simulink model "case2"  (R2024b)
settings: Solver=FixedStepAuto  StartTime=0  StopTime=1  FixedStep=1e-7  RelTol=1e-3
values from neighbouring files (symbols this model uses):
  SG_D_1_D = 0.01056    [IEEE9_case_parameters.m]    (also in case1_parameters.m; case2_parameters.m; case3_parameters.m; case4_parameters.m)
  SG_D_1_EnableSaturation = 0    [IEEE9_case_parameters.m]    (also in case1_parameters.m; case2_parameters.m; case3_parameters.m; case4_parameters.m)
  SG_D_1_f0 = 60    [IEEE9_case_parameters.m]    (also in case1_parameters.m; case2_parameters.m; case3_parameters.m; case4_parameters.m)
  SG_D_1_H = 7.5    [IEEE9_case_parameters.m]    (also in case1_parameters.m; case2_parameters.m; case3_parameters.m; case4_parameters.m)
  SG_D_1_K_A = 20    [IEEE9_case_parameters.m]    (also in case1_parameters.m; case2_parameters.m; case3_parameters.m; case4_parameters.m)
  SG_D_1_K_E = 1.000000e+1    (= 10)    [IEEE9_case_parameters.m]    (also in case1_parameters.m; case2_parameters.m; case3_parameters.m; case4_parameters.m)
  SG_D_1_K_F = 2.363    [IEEE9_case_parameters.m]    (also in case1_parameters.m; case2_parameters.m; case3_parameters.m; case4_parameters.m)
  SG_D_1_K_s = 0.5    [IEEE9_case_parameters.m]    (also in case1_parameters.m = 5; case2_parameters.m = 5; case3_parameters.m = 5; case4_parameters.m = 5)
  SG_D_1_R_a = 0.001088    [IEEE9_case_parameters.m]    (also in case1_parameters.m; case2_parameters.m; case3_parameters.m; case4_parameters.m)
  SG_D_1_S_A = 1    [IEEE9_case_parameters.m]    (also in case1_parameters.m; case2_parameters.m; case3_parameters.m; case4_parameters.m)
  SG_D_1_S_B = 0.103    [IEEE9_case_parameters.m]    (also in case1_parameters.m; case2_parameters.m; case3_parameters.m; case4_parameters.m)
  SG_D_1_S_N = 10.659857    [IEEE9_case_parameters.m]    (also in case1_parameters.m; case2_parameters.m; case3_parameters.m; case4_parameters.m)
  SG_D_1_SpeedPara = 200    [IEEE9_case_parameters.m]    (also in case1_parameters.m; case2_parameters.m; case3_parameters.m; case4_parameters.m)
  SG_D_1_T_0 = 0.720173    [IEEE9_case_parameters.m]    (also in case1_parameters.m = 0.755522; case2_parameters.m = 0.808931; case3_parameters.m = 0.869402; case4_parameters.m = 0.729316)
  SG_D_1_T_1 = 0.3    [IEEE9_case_parameters.m]    (also in case1_parameters.m; case2_parameters.m; case3_parameters.m; case4_parameters.m)
  SG_D_1_T_2 = 0.05    [IEEE9_case_parameters.m]    (also in case1_parameters.m; case2_parameters.m; case3_parameters.m; case4_parameters.m)
  SG_D_1_T_3 = 0.02    [IEEE9_case_parameters.m]    (also in case1_parameters.m; case2_parameters.m; case3_parameters.m; case4_parameters.m)
  SG_D_1_T_4 = 0.005    [IEEE9_case_parameters.m]    (also in case1_parameters.m; case2_parameters.m; case3_parameters.m; case4_parameters.m)
  SG_D_1_T_A = 0.02    [IEEE9_case_parameters.m]    (also in case1_parameters.m; case2_parameters.m; case3_parameters.m; case4_parameters.m)
  SG_D_1_T_dd = 8.000000e+0    (= 8)    [IEEE9_case_parameters.m]    (also in case1_parameters.m; case2_parameters.m; case3_parameters.m; case4_parameters.m)
  SG_D_1_T_ddd = 0.04    [IEEE9_case_parameters.m]    (also in case1_parameters.m; case2_parameters.m; case3_parameters.m; case4_parameters.m)
  SG_D_1_T_E = 0.314    [IEEE9_case_parameters.m]    (also in case1_parameters.m; case2_parameters.m; case3_parameters.m; case4_parameters.m)
  SG_D_1_T_F = 0.35    [IEEE9_case_parameters.m]    (also in case1_parameters.m; case2_parameters.m; case3_parameters.m; case4_parameters.m)
  SG_D_1_T_qd = 0.8    [IEEE9_case_parameters.m]    (also in case1_parameters.m; case2_parameters.m; case3_parameters.m; case4_parameters.m)
  SG_D_1_T_qdd = 0.02    [IEEE9_case_parameters.m]    (also in case1_parameters.m; case2_parameters.m; case3_parameters.m; case4_parameters.m)
  SG_D_1_T_speed = 0.1    [IEEE9_case_parameters.m]    (also in case1_parameters.m = 200; case2_parameters.m = 200; case3_parameters.m = 200; case4_parameters.m = 200)
  SG_D_1_T_w = 0.5    [IEEE9_case_parameters.m]    (also in case1_parameters.m; case2_parameters.m; case3_parameters.m; case4_parameters.m)
  SG_D_1_V_ref = 1.990276    [IEEE9_case_parameters.m]    (also in case1_parameters.m = 2.042296; case2_parameters.m = 2.051388; case3_parameters.m = 2.089584; case4_parameters.m = 2.01845)
  SG_D_1_w_ref = 376.991118    [IEEE9_case_parameters.m]    (also in case1_parameters.m; case2_parameters.m; case3_parameters.m; case4_parameters.m)
  SG_D_1_wb = 6.000000e+1    (= 60)    [IEEE9_case_parameters.m]    (also in case1_parameters.m; case2_parameters.m; case3_parameters.m; case4_parameters.m)
  SG_D_1_x_d = 1.9    [IEEE9_case_parameters.m]    (also in case1_parameters.m; case2_parameters.m; case3_parameters.m; case4_parameters.m)
  SG_D_1_x_dd = 0.302    [IEEE9_case_parameters.m]    (also in case1_parameters.m; case2_parameters.m; case3_parameters.m; case4_parameters.m)
  SG_D_1_x_ddd = 0.204    [IEEE9_case_parameters.m]    (also in case1_parameters.m; case2_parameters.m; case3_parameters.m; case4_parameters.m)
  SG_D_1_x_l = 0.05    [IEEE9_case_parameters.m]    (also in case1_parameters.m; case2_parameters.m; case3_parameters.m; case4_parameters.m)
  SG_D_1_x_q = 1.3    [IEEE9_case_parameters.m]    (also in case1_parameters.m; case2_parameters.m; case3_parameters.m; case4_parameters.m)
  SG_D_1_x_qd = 0.5    [IEEE9_case_parameters.m]    (also in case1_parameters.m; case2_parameters.m; case3_parameters.m; case4_parameters.m)
  SG_D_1_x_qdd = 0.3    [IEEE9_case_parameters.m]    (also in case1_parameters.m; case2_parameters.m; case3_parameters.m; case4_parameters.m)
  SG_D_2_D = 0.02    [IEEE9_case_parameters.m]    (also in case1_parameters.m; case2_parameters.m; case3_parameters.m; case4_parameters.m)
  SG_D_2_EnableSaturation = 0    [IEEE9_case_parameters.m]    (also in case1_parameters.m; case2_parameters.m; case3_parameters.m; case4_parameters.m)
  SG_D_2_f0 = 60    [IEEE9_case_parameters.m]    (also in case1_parameters.m; case2_parameters.m; case3_parameters.m; case4_parameters.m)
  SG_D_2_H = 8.000000e+0    (= 8)    [IEEE9_case_parameters.m]    (also in case1_parameters.m; case2_parameters.m; case3_parameters.m; case4_parameters.m)
  SG_D_2_K_A = 20    [IEEE9_case_parameters.m]    (also in case1_parameters.m; case2_parameters.m; case3_parameters.m; case4_parameters.m)
  SG_D_2_K_E = 1.000000e+1    (= 10)    [IEEE9_case_parameters.m]    (also in case1_parameters.m; case2_parameters.m; case3_parameters.m; case4_parameters.m)
  SG_D_2_K_F = 2.363    [IEEE9_case_parameters.m]    (also in case1_parameters.m; case2_parameters.m; case3_parameters.m; case4_parameters.m)
  SG_D_2_K_s = 0.5    [IEEE9_case_parameters.m]    (also in case1_parameters.m = 4; case2_parameters.m = 4; case3_parameters.m = 4; case4_parameters.m = 4)
  SG_D_2_R_a = 0.001088    [IEEE9_case_parameters.m]    (also in case1_parameters.m; case2_parameters.m; case3_parameters.m; case4_parameters.m)
  SG_D_2_S_A = 1    [IEEE9_case_parameters.m]    (also in case1_parameters.m; case2_parameters.m; case3_parameters.m; case4_parameters.m)
  SG_D_2_S_B = 0.103    [IEEE9_case_parameters.m]    (also in case1_parameters.m; case2_parameters.m; case3_parameters.m; case4_parameters.m)
  SG_D_2_S_N = 10.659857    [IEEE9_case_parameters.m]    (also in case1_parameters.m; case2_parameters.m; case3_parameters.m; case4_parameters.m)
  SG_D_2_SpeedPara = 200    [IEEE9_case_parameters.m]    (also in case1_parameters.m; case2_parameters.m; case3_parameters.m; case4_parameters.m)
  SG_D_2_T_0 = 1.632913    [IEEE9_case_parameters.m]    (also in case1_parameters.m = 1.632925; case2_parameters.m = 1.632915; case3_parameters.m = 1.632914; case4_parameters.m = 1.632927)
  SG_D_2_T_1 = 0.2    [IEEE9_case_parameters.m]    (also in case1_parameters.m; case2_parameters.m; case3_parameters.m; case4_parameters.m)
  SG_D_2_T_2 = 0.05    [IEEE9_case_parameters.m]    (also in case1_parameters.m; case2_parameters.m; case3_parameters.m; case4_parameters.m)
  SG_D_2_T_3 = 0.02    [IEEE9_case_parameters.m]    (also in case1_parameters.m; case2_parameters.m; case3_parameters.m; case4_parameters.m)
  SG_D_2_T_4 = 0.005    [IEEE9_case_parameters.m]    (also in case1_parameters.m; case2_parameters.m; case3_parameters.m; case4_parameters.m)
  SG_D_2_T_A = 0.02    [IEEE9_case_parameters.m]    (also in case1_parameters.m; case2_parameters.m; case3_parameters.m; case4_parameters.m)
  SG_D_2_T_dd = 7.9    [IEEE9_case_parameters.m]    (also in case1_parameters.m; case2_parameters.m; case3_parameters.m; case4_parameters.m)
  SG_D_2_T_ddd = 0.04    [IEEE9_case_parameters.m]    (also in case1_parameters.m; case2_parameters.m; case3_parameters.m; case4_parameters.m)
  SG_D_2_T_E = 0.314    [IEEE9_case_parameters.m]    (also in case1_parameters.m; case2_parameters.m; case3_parameters.m; case4_parameters.m)
  SG_D_2_T_F = 0.35    [IEEE9_case_parameters.m]    (also in case1_parameters.m; case2_parameters.m; case3_parameters.m; case4_parameters.m)
  SG_D_2_T_qd = 0.8    [IEEE9_case_parameters.m]    (also in case1_parameters.m; case2_parameters.m; case3_parameters.m; case4_parameters.m)
  SG_D_2_T_qdd = 0.015    [IEEE9_case_parameters.m]    (also in case1_parameters.m; case2_parameters.m; case3_parameters.m; case4_parameters.m)
  SG_D_2_T_speed = 0.1    [IEEE9_case_parameters.m]    (also in case1_parameters.m = 150; case2_parameters.m = 150; case3_parameters.m = 150; case4_parameters.m = 150)
  SG_D_2_T_w = 0.35    [IEEE9_case_parameters.m]    (also in case1_parameters.m; case2_parameters.m; case3_parameters.m; case4_parameters.m)
  SG_D_2_V_ref = 2.58547    [IEEE9_case_parameters.m]    (also in case1_parameters.m = 2.597896; case2_parameters.m = 2.587136; case3_parameters.m = 2.586042; case4_parameters.m = 2.599679)
  SG_D_2_w_ref = 376.991118    [IEEE9_case_parameters.m]    (also in case1_parameters.m; case2_parameters.m; case3_parameters.m; case4_parameters.m)
  SG_D_2_wb = 6.000000e+1    (= 60)    [IEEE9_case_parameters.m]    (also in case1_parameters.m; case2_parameters.m; case3_parameters.m; case4_parameters.m)
  SG_D_2_x_d = 1.8    [IEEE9_case_parameters.m]    (also in case1_parameters.m; case2_parameters.m; case3_parameters.m; case4_parameters.m)
  SG_D_2_x_dd = 0.302    [IEEE9_case_parameters.m]    (also in case1_parameters.m; case2_parameters.m; case3_parameters.m; case4_parameters.m)
  SG_D_2_x_ddd = 0.204    [IEEE9_case_parameters.m]    (also in case1_parameters.m; case2_parameters.m; case3_parameters.m; case4_parameters.m)
  SG_D_2_x_l = 0.05    [IEEE9_case_parameters.m]    (also in case1_parameters.m; case2_parameters.m; case3_parameters.m; case4_parameters.m)
  SG_D_2_x_q = 1.25    [IEEE9_case_parameters.m]    (also in case1_parameters.m; case2_parameters.m; case3_parameters.m; case4_parameters.m)
  SG_D_2_x_qd = 0.5    [IEEE9_case_parameters.m]    (also in case1_parameters.m; case2_parameters.m; case3_parameters.m; case4_parameters.m)
  SG_D_2_x_qdd = 0.3    [IEEE9_case_parameters.m]    (also in case1_parameters.m; case2_parameters.m; case3_parameters.m; case4_parameters.m)
  SG_D_3_D = 0.02    [IEEE9_case_parameters.m]    (also in case1_parameters.m; case2_parameters.m; case3_parameters.m; case4_parameters.m)
  SG_D_3_EnableSaturation = 0    [IEEE9_case_parameters.m]    (also in case1_parameters.m; case2_parameters.m; case3_parameters.m; case4_parameters.m)
  SG_D_3_f0 = 60    [IEEE9_case_parameters.m]    (also in case1_parameters.m; case2_parameters.m; case3_parameters.m; case4_parameters.m)
  SG_D_3_H = 7.7    [IEEE9_case_parameters.m]    (also in case1_parameters.m; case2_parameters.m; case3_parameters.m; case4_parameters.m)
  SG_D_3_K_A = 20    [IEEE9_case_parameters.m]    (also in case1_parameters.m; case2_parameters.m; case3_parameters.m; case4_parameters.m)
  SG_D_3_K_E = 1.000000e+1    (= 10)    [IEEE9_case_parameters.m]    (also in case1_parameters.m; case2_parameters.m; case3_parameters.m; case4_parameters.m)
  SG_D_3_K_F = 2.363    [IEEE9_case_parameters.m]    (also in case1_parameters.m; case2_parameters.m; case3_parameters.m; case4_parameters.m)
  SG_D_3_K_s = 0.2    [IEEE9_case_parameters.m]    (also in case1_parameters.m = 2; case2_parameters.m = 2; case3_parameters.m = 2; case4_parameters.m = 2)
  SG_D_3_R_a = 0.001088    [IEEE9_case_parameters.m]    (also in case1_parameters.m; case2_parameters.m; case3_parameters.m; case4_parameters.m)
  SG_D_3_S_A = 1    [IEEE9_case_parameters.m]    (also in case1_parameters.m; case2_parameters.m; case3_parameters.m; case4_parameters.m)
  SG_D_3_S_B = 0.103    [IEEE9_case_parameters.m]    (also in case1_parameters.m; case2_parameters.m; case3_parameters.m; case4_parameters.m)
  SG_D_3_S_N = 10.659857    [IEEE9_case_parameters.m]    (also in case1_parameters.m; case2_parameters.m; case3_parameters.m; case4_parameters.m)
  SG_D_3_SpeedPara = 200    [IEEE9_case_parameters.m]    (also in case1_parameters.m; case2_parameters.m; case3_parameters.m; case4_parameters.m)
  SG_D_3_T_0 = 0.850788    [IEEE9_case_parameters.m]    (also in case1_parameters.m = 0.850786; case2_parameters.m = 0.850787; case3_parameters.m; case4_parameters.m = 0.850786)
  SG_D_3_T_1 = 0.2    [IEEE9_case_parameters.m]    (also in case1_parameters.m; case2_parameters.m; case3_parameters.m; case4_parameters.m)
  SG_D_3_T_2 = 0.05    [IEEE9_case_parameters.m]    (also in case1_parameters.m; case2_parameters.m; case3_parameters.m; case4_parameters.m)
  SG_D_3_T_3 = 0.02    [IEEE9_case_parameters.m]    (also in case1_parameters.m; case2_parameters.m; case3_parameters.m; case4_parameters.m)
  SG_D_3_T_4 = 0.005    [IEEE9_case_parameters.m]    (also in case1_parameters.m; case2_parameters.m; case3_parameters.m; case4_parameters.m)
  SG_D_3_T_A = 0.02    [IEEE9_case_parameters.m]    (also in case1_parameters.m; case2_parameters.m; case3_parameters.m; case4_parameters.m)
  SG_D_3_T_dd = 8.1    [IEEE9_case_parameters.m]    (also in case1_parameters.m; case2_parameters.m; case3_parameters.m; case4_parameters.m)
  SG_D_3_T_ddd = 0.04    [IEEE9_case_parameters.m]    (also in case1_parameters.m; case2_parameters.m; case3_parameters.m; case4_parameters.m)
  SG_D_3_T_E = 0.314    [IEEE9_case_parameters.m]    (also in case1_parameters.m; case2_parameters.m; case3_parameters.m; case4_parameters.m)
  SG_D_3_T_F = 0.35    [IEEE9_case_parameters.m]    (also in case1_parameters.m; case2_parameters.m; case3_parameters.m; case4_parameters.m)
  SG_D_3_T_qd = 0.8    [IEEE9_case_parameters.m]    (also in case1_parameters.m; case2_parameters.m; case3_parameters.m; case4_parameters.m)
  SG_D_3_T_qdd = 0.015    [IEEE9_case_parameters.m]    (also in case1_parameters.m; case2_parameters.m; case3_parameters.m; case4_parameters.m)
  SG_D_3_T_speed = 0.1    [IEEE9_case_parameters.m]    (also in case1_parameters.m = 180; case2_parameters.m = 180; case3_parameters.m = 180; case4_parameters.m = 180)
  SG_D_3_T_w = 0.4    [IEEE9_case_parameters.m]    (also in case1_parameters.m; case2_parameters.m; case3_parameters.m; case4_parameters.m)
  SG_D_3_V_ref = 1.892727    [IEEE9_case_parameters.m]    (also in case1_parameters.m = 1.906439; case2_parameters.m = 1.895535; case3_parameters.m = 1.892105; case4_parameters.m = 1.906598)
  SG_D_3_w_ref = 376.991118    [IEEE9_case_parameters.m]    (also in case1_parameters.m; case2_parameters.m; case3_parameters.m; case4_parameters.m)
  SG_D_3_wb = 6.000000e+1    (= 60)    [IEEE9_case_parameters.m]    (also in case1_parameters.m; case2_parameters.m; case3_parameters.m; case4_parameters.m)
  SG_D_3_x_d = 1.85    [IEEE9_case_parameters.m]    (also in case1_parameters.m; case2_parameters.m; case3_parameters.m; case4_parameters.m)
  SG_D_3_x_dd = 0.302    [IEEE9_case_parameters.m]    (also in case1_parameters.m; case2_parameters.m; case3_parameters.m; case4_parameters.m)
  SG_D_3_x_ddd = 0.204    [IEEE9_case_parameters.m]    (also in case1_parameters.m; case2_parameters.m; case3_parameters.m; case4_parameters.m)
  SG_D_3_x_l = 0.05    [IEEE9_case_parameters.m]    (also in case1_parameters.m; case2_parameters.m; case3_parameters.m; case4_parameters.m)
  SG_D_3_x_q = 1.2    [IEEE9_case_parameters.m]    (also in case1_parameters.m; case2_parameters.m; case3_parameters.m; case4_parameters.m)
  SG_D_3_x_qd = 0.5    [IEEE9_case_parameters.m]    (also in case1_parameters.m; case2_parameters.m; case3_parameters.m; case4_parameters.m)
  SG_D_3_x_qdd = 0.3    [IEEE9_case_parameters.m]    (also in case1_parameters.m; case2_parameters.m; case3_parameters.m; case4_parameters.m)
(part 1 of 12)
settings Model: Creator=Greg  LastModifiedBy=Greg

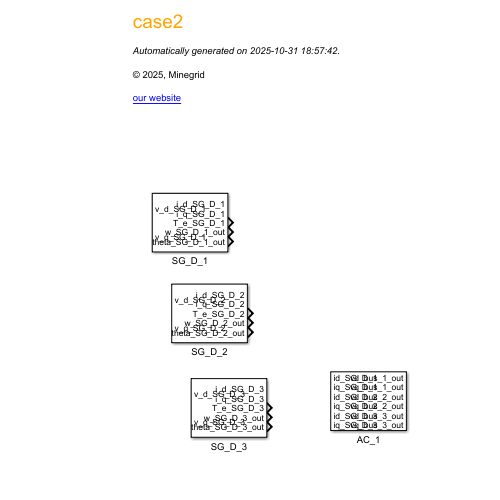
[thumbnail: Simulink's stored preview of the top-level diagram]
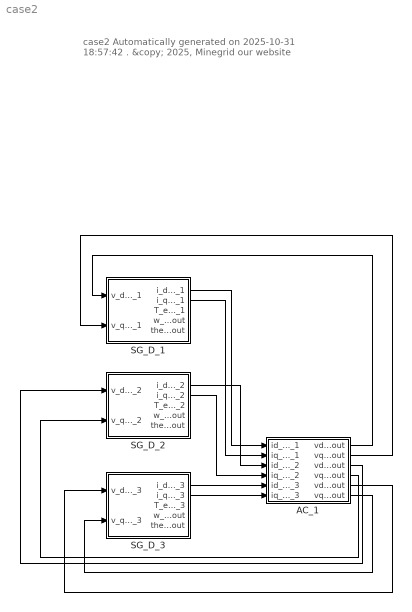
== system case2 ==
  note: case2
      | Automatically generated on 2025-10-31 18:57:42 .
      | &copy; 2025, Minegrid
      | our website
  AC_1 : Subsystem  mask(AC_1){}
      mask help: Parameters Interface of AC_1
  SG_D_1 : Subsystem  mask(SG_D_1){T_0=SG_D_1_T_0, w_ref=SG_D_1_w_ref, V_ref=SG_D_1_V_ref, x_d=SG_D_1_x_d, x_dd=SG_D_1_x_dd, x_ddd=SG_D_1_x_ddd, x_q=SG_D_1_x_q, x_qd=SG_D_1_x_qd, x_qdd=SG_D_1_x_qdd, x_l=SG_D_1_x_l, R_a=SG_D_1_R_a, T_dd=SG_D_1_T_dd, T_ddd=SG_D_1_T_ddd, T_qd=SG_D_1_T_qd, T_qdd=SG_D_1_T_qdd, H=SG_D_1_H, D=SG_D_1_D, SpeedPara=SG_D_1_SpeedPara, K_A=SG_D_1_K_A, EnableSaturation=SG_D_1_EnableSaturation, f0=SG_D_1_f0, T_speed=SG_D_1_T_speed, T_E=SG_D_1_T_E, T_A=SG_D_1_T_A, T_F=SG_D_1_T_F, K_E=SG_D_1_K_E, K_F=SG_D_1_K_F, K_s=SG_D_1_K_s, T_1=SG_D_1_T_1, T_2=SG_D_1_T_2, T_3=SG_D_1_T_3, T_4=SG_D_1_T_4, T_w=SG_D_1_T_w, wb=SG_D_1_wb, S_A=SG_D_1_S_A, S_B=SG_D_1_S_B, S_N=SG_D_1_S_N}
      mask help: Parameters Interface of SG_D_1
  SG_D_2 : Subsystem  mask(SG_D_2){T_0=SG_D_2_T_0, w_ref=SG_D_2_w_ref, V_ref=SG_D_2_V_ref, x_d=SG_D_2_x_d, x_dd=SG_D_2_x_dd, x_ddd=SG_D_2_x_ddd, x_q=SG_D_2_x_q, x_qd=SG_D_2_x_qd, x_qdd=SG_D_2_x_qdd, x_l=SG_D_2_x_l, R_a=SG_D_2_R_a, T_dd=SG_D_2_T_dd, T_ddd=SG_D_2_T_ddd, T_qd=SG_D_2_T_qd, T_qdd=SG_D_2_T_qdd, H=SG_D_2_H, D=SG_D_2_D, SpeedPara=SG_D_2_SpeedPara, K_A=SG_D_2_K_A, EnableSaturation=SG_D_2_EnableSaturation, f0=SG_D_2_f0, T_speed=SG_D_2_T_speed, T_E=SG_D_2_T_E, T_A=SG_D_2_T_A, T_F=SG_D_2_T_F, K_E=SG_D_2_K_E, K_F=SG_D_2_K_F, K_s=SG_D_2_K_s, T_1=SG_D_2_T_1, T_2=SG_D_2_T_2, T_3=SG_D_2_T_3, T_4=SG_D_2_T_4, T_w=SG_D_2_T_w, wb=SG_D_2_wb, S_A=SG_D_2_S_A, S_B=SG_D_2_S_B, S_N=SG_D_2_S_N}
      mask help: Parameters Interface of SG_D_2
  SG_D_3 : Subsystem  mask(SG_D_3){T_0=SG_D_3_T_0, w_ref=SG_D_3_w_ref, V_ref=SG_D_3_V_ref, x_d=SG_D_3_x_d, x_dd=SG_D_3_x_dd, x_ddd=SG_D_3_x_ddd, x_q=SG_D_3_x_q, x_qd=SG_D_3_x_qd, x_qdd=SG_D_3_x_qdd, x_l=SG_D_3_x_l, R_a=SG_D_3_R_a, T_dd=SG_D_3_T_dd, T_ddd=SG_D_3_T_ddd, T_qd=SG_D_3_T_qd, T_qdd=SG_D_3_T_qdd, H=SG_D_3_H, D=SG_D_3_D, SpeedPara=SG_D_3_SpeedPara, K_A=SG_D_3_K_A, EnableSaturation=SG_D_3_EnableSaturation, f0=SG_D_3_f0, T_speed=SG_D_3_T_speed, T_E=SG_D_3_T_E, T_A=SG_D_3_T_A, T_F=SG_D_3_T_F, K_E=SG_D_3_K_E, K_F=SG_D_3_K_F, K_s=SG_D_3_K_s, T_1=SG_D_3_T_1, T_2=SG_D_3_T_2, T_3=SG_D_3_T_3, T_4=SG_D_3_T_4, T_w=SG_D_3_T_w, wb=SG_D_3_wb, S_A=SG_D_3_S_A, S_B=SG_D_3_S_B, S_N=SG_D_3_S_N}
      mask help: Parameters Interface of SG_D_3
  wires:
  SG_D_2/2(i_q_SG_D_2) -> AC_1/4(iq_SG_D_2)
  SG_D_1/2(i_q_SG_D_1) -> AC_1/2(iq_SG_D_1)
  SG_D_1/1(i_d_SG_D_1) -> AC_1/1(id_SG_D_1)
  SG_D_2/1(i_d_SG_D_2) -> AC_1/3(id_SG_D_2)
  AC_1/1(vd_bus_1_out) -> SG_D_1/1(v_d_SG_D_1)
  SG_D_3/1(i_d_SG_D_3) -> AC_1/5(id_SG_D_3)
  AC_1/2(vq_bus_1_out) -> SG_D_1/2(v_q_SG_D_1)
  SG_D_3/2(i_q_SG_D_3) -> AC_1/6(iq_SG_D_3)
  AC_1/3(vd_bus_2_out) -> SG_D_2/1(v_d_SG_D_2)
  AC_1/4(vq_bus_2_out) -> SG_D_2/2(v_q_SG_D_2)
  AC_1/5(vd_bus_3_out) -> SG_D_3/1(v_d_SG_D_3)
  AC_1/6(vq_bus_3_out) -> SG_D_3/2(v_q_SG_D_3)

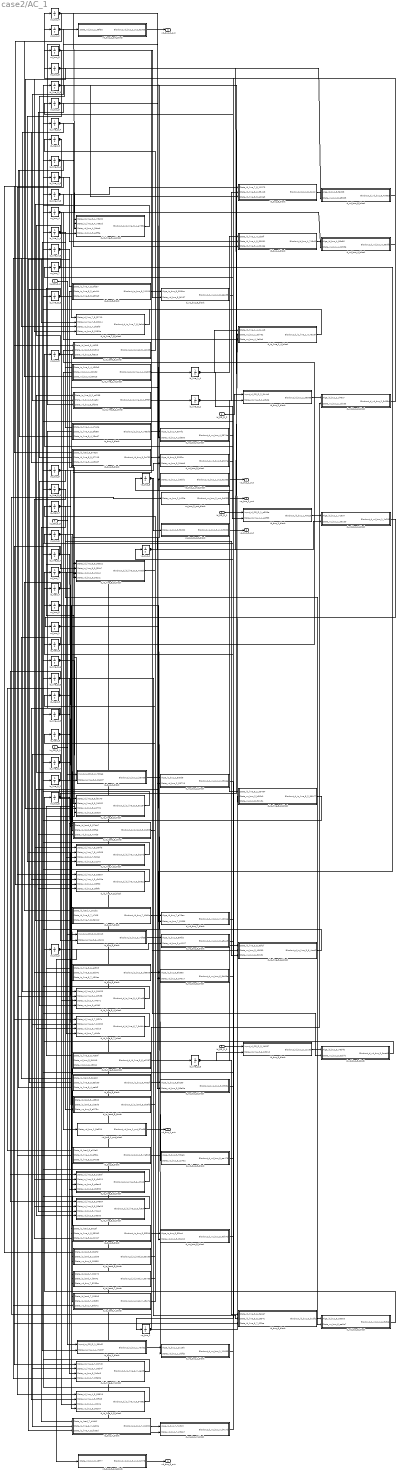
== system case2/AC_1 ==
  id_SG_D_1 : Inport
  iq_SG_D_1 : Inport  Port=2
  id_SG_D_2 : Inport  Port=3
  iq_SG_D_2 : Inport  Port=4
  id_SG_D_3 : Inport  Port=5
  iq_SG_D_3 : Inport  Port=6
  d_id_line_1_4_block : Subsystem
  d_id_line_3_6_block : Subsystem
  d_id_line_4_5_block : Subsystem
  d_id_line_5_6_block : Subsystem
  d_id_line_6_7_block : Subsystem
  d_id_line_7_8_block : Subsystem
  d_id_line_8_2_block : Subsystem
  d_id_line_8_9_block : Subsystem
  d_id_line_9_4_block : Subsystem
  d_id_load_5_block : Subsystem
  d_id_load_7_block : Subsystem
  d_id_load_9_block : Subsystem
  d_iq_line_1_4_block : Subsystem
  d_iq_line_3_6_block : Subsystem
  d_iq_line_4_5_block : Subsystem
  d_iq_line_5_6_block : Subsystem
  d_iq_line_6_7_block : Subsystem
  d_iq_line_7_8_block : Subsystem
  d_iq_line_8_2_block : Subsystem
  d_iq_line_8_9_block : Subsystem
  d_iq_line_9_4_block : Subsystem
  d_iq_load_5_block : Subsystem
  d_iq_load_7_block : Subsystem
  d_iq_load_9_block : Subsystem
  d_vd_bus_1_block : Subsystem
  d_vd_bus_2_block : Subsystem
  d_vd_bus_3_block : Subsystem
  d_vd_bus_4_block : Subsystem
  d_vd_bus_5_block : Subsystem
  d_vd_bus_6_block : Subsystem
  d_vd_bus_7_block : Subsystem
  d_vd_bus_8_block : Subsystem
  d_vd_bus_9_block : Subsystem
  d_vq_bus_1_block : Subsystem
  d_vq_bus_2_block : Subsystem
  d_vq_bus_3_block : Subsystem
  d_vq_bus_4_block : Subsystem
  d_vq_bus_5_block : Subsystem
  d_vq_bus_6_block : Subsystem
  d_vq_bus_7_block : Subsystem
  d_vq_bus_8_block : Subsystem
  d_vq_bus_9_block : Subsystem
  id_bus_1_block : Subsystem
  id_bus_2_block : Subsystem
  id_bus_3_block : Subsystem
  id_bus_4_block : Subsystem
  id_bus_5_block : Subsystem
  id_bus_6_block : Subsystem
  id_bus_7_block : Subsystem
  id_bus_8_block : Subsystem
  id_bus_9_block : Subsystem
  id_line_1_4 : Integrator  InitialCondition=0.8082
  id_line_3_6 : Integrator  InitialCondition=0.8457
  id_line_4_5 : Integrator  InitialCondition=0.3479
  id_line_5_6 : Integrator  InitialCondition=-0.5937
  id_line_6_7 : Integrator  InitialCondition=0.2581
  id_line_7_8 : Integrator  InitialCondition=-0.7857
  id_line_8_2 : Integrator  InitialCondition=-1.6336
  id_line_8_9 : Integrator  InitialCondition=0.8599
  id_line_9_4 : Integrator  InitialCondition=-0.4527
  id_load_5 : Integrator  InitialCondition=0.9220949046655532
  id_load_7 : Integrator  InitialCondition=1.043451181339317
  id_load_9 : Integrator  InitialCondition=1.2932545562048015
  iq_bus_1_block : Subsystem
  iq_bus_2_block : Subsystem
  iq_bus_3_block : Subsystem
  iq_bus_4_block : Subsystem
  iq_bus_5_block : Subsystem
  iq_bus_6_block : Subsystem
  iq_bus_7_block : Subsystem
  iq_bus_8_block : Subsystem
  iq_bus_9_block : Subsystem
  iq_line_1_4 : Integrator  InitialCondition=-0.2445
  iq_line_3_6 : Integrator  InitialCondition=0.0905
  iq_line_4_5 : Integrator  InitialCondition=-0.0855
  iq_line_5_6 : Integrator  InitialCondition=0.0474
  iq_line_6_7 : Integrator  InitialCondition=-0.1464
  iq_line_7_8 : Integrator  InitialCondition=0.0394
  iq_line_8_2 : Integrator  InitialCondition=-0.1018
  iq_line_8_9 : Integrator  InitialCondition=-0.0851
  iq_line_9_4 : Integrator  InitialCondition=0.3237
  iq_load_5 : Integrator  InitialCondition=-0.3839325127306236
  iq_load_7 : Integrator  InitialCondition=-0.3621433932821941
  iq_load_9 : Integrator  InitialCondition=-0.6389217940515789
  vd_bus_1 : Integrator  InitialCondition=1.0
  vd_bus_1_out_block : Subsystem
  vd_bus_2 : Integrator  InitialCondition=0.9882467673333026
  vd_bus_2_out_block : Subsystem
  vd_bus_3 : Integrator  InitialCondition=0.9975390275639218
  vd_bus_3_out_block : Subsystem
  vd_bus_4 : Integrator  InitialCondition=0.9862000078347533
  vd_bus_5 : Integrator  InitialCondition=0.9728788660812012
  vd_bus_6 : Integrator  InitialCondition=1.0027357442532745
  vd_bus_7 : Integrator  InitialCondition=0.9853647003996387
  vd_bus_8 : Integrator  InitialCondition=0.9944780823647019
  vd_bus_9 : Integrator  InitialCondition=0.9549499810613831
  vq_bus_1 : Integrator  InitialCondition=0.0
  vq_bus_1_out_block : Subsystem
  vq_bus_2 : Integrator  InitialCondition=0.1528670234395801
  vq_bus_2_out_block : Subsystem
  vq_bus_3 : Integrator  InitialCondition=0.07011339734191536
  vq_bus_3_out_block : Subsystem
  vq_bus_4 : Integrator  InitialCondition=-0.04560902069175053
  vq_bus_5 : Integrator  InitialCondition=-0.07558645534686588
  vq_bus_6 : Integrator  InitialCondition=0.021554874164418644
  vq_bus_7 : Integrator  InitialCondition=-0.002285093510706759
  vq_bus_8 : Integrator  InitialCondition=0.05282760910237743
  vq_bus_9 : Integrator  InitialCondition=-0.08023822590177464
  vd_bus_1_out : Outport
  vq_bus_1_out : Outport  Port=2
  vd_bus_2_out : Outport  Port=3
  vq_bus_2_out : Outport  Port=4
  vd_bus_3_out : Outport  Port=5
  vq_bus_3_out : Outport  Port=6
  wires:
  iq_SG_D_2/1 -> iq_bus_2_block/1(Input_iq_SG_D_2_708e6)
  id_bus_4_block/1(Blockout_id_bus_4_748d0) -> d_vd_bus_4_block/1(Alge_id_bus_4_86c66)
  vd_bus_1_out_block/1(Blockout_vd_bus_1_out_57e66) -> vd_bus_1_out/1
  vq_bus_1_out_block/1(Blockout_vq_bus_1_out_5135a) -> vq_bus_1_out/1
  id_load_9/1 -> d_id_load_9_block/1(State_id_load_9_4df15), id_bus_9_block/1(State_id_load_9_97526), d_iq_load_9_block/1(State_id_load_9_3b2fd)
  vq_bus_2_out_block/1(Blockout_vq_bus_2_out_0c630) -> vq_bus_2_out/1
  d_id_line_1_4_block/1(Blockout_d_id_line_1_4_0ab3f) -> id_line_1_4/1
  iq_SG_D_3/1 -> iq_bus_3_block/1(Input_iq_SG_D_3_22043)
  vq_bus_1/1 -> d_vd_bus_1_block/2(State_vq_bus_1_a61e0), vq_bus_1_out_block/1(State_vq_bus_1_b3dd1), d_iq_line_1_4_block/2(State_vq_bus_1_ed792)
  vd_bus_3_out_block/1(Blockout_vd_bus_3_out_24978) -> vd_bus_3_out/1
  d_vd_bus_4_block/1(Blockout_d_vd_bus_4_39df0) -> vd_bus_4/1
  d_iq_line_8_2_block/1(Blockout_d_iq_line_8_2_96b77) -> iq_line_8_2/1
  id_SG_D_3/1 -> id_bus_3_block/1(Input_id_SG_D_3_1b557)
  id_bus_9_block/1(Blockout_id_bus_9_2e79f) -> d_vd_bus_9_block/1(Alge_id_bus_9_3932a)
  iq_SG_D_1/1 -> iq_bus_1_block/1(Input_iq_SG_D_1_56b6f)
  iq_bus_2_block/1(Blockout_iq_bus_2_b5069) -> d_vq_bus_2_block/1(Alge_iq_bus_2_5c6d8)
  vd_bus_6/1 -> d_vq_bus_6_block/2(State_vd_bus_6_e4a17), d_id_line_3_6_block/3(State_vd_bus_6_1884c), d_id_line_6_7_block/3(State_vd_bus_6_7ad19), d_id_line_5_6_block/4(State_vd_bus_6_a9a0a)
  d_id_line_4_5_block/1(Blockout_d_id_line_4_5_ba811) -> id_line_4_5/1
  vq_bus_2/1 -> d_iq_line_8_2_block/2(State_vq_bus_2_b36b0), d_vd_bus_2_block/2(State_vq_bus_2_1d16a), vq_bus_2_out_block/1(State_vq_bus_2_b12fe)
  id_SG_D_2/1 -> id_bus_2_block/1(Input_id_SG_D_2_544c5)
  id_SG_D_1/1 -> id_bus_1_block/1(Input_id_SG_D_1_a599e)
  iq_bus_4_block/1(Blockout_iq_bus_4_79ed0) -> d_vq_bus_4_block/1(Alge_iq_bus_4_697f2)
  id_line_6_7/1 -> d_id_line_6_7_block/1(State_id_line_6_7_5f97c), d_iq_line_6_7_block/1(State_id_line_6_7_327c8), id_bus_6_block/3(State_id_line_6_7_02fca), id_bus_7_block/2(State_id_line_6_7_c74f6)
  id_bus_2_block/1(Blockout_id_bus_2_a8585) -> d_vd_bus_2_block/1(Alge_id_bus_2_d46c7)
  vq_bus_7/1 -> d_vd_bus_7_block/2(State_vq_bus_7_81f66), d_iq_line_7_8_block/3(State_vq_bus_7_5bef0), d_iq_line_6_7_block/4(State_vq_bus_7_35686), d_iq_load_7_block/3(State_vq_bus_7_90b72)
  vd_bus_2_out_block/1(Blockout_vd_bus_2_out_3230a) -> vd_bus_2_out/1
  iq_bus_9_block/1(Blockout_iq_bus_9_46ecf) -> d_vq_bus_9_block/1(Alge_iq_bus_9_5bc50)
  vq_bus_3_out_block/1(Blockout_vq_bus_3_out_fc8db) -> vq_bus_3_out/1
  iq_bus_8_block/1(Blockout_iq_bus_8_11109) -> d_vq_bus_8_block/1(Alge_iq_bus_8_0994e)
  d_id_line_6_7_block/1(Blockout_d_id_line_6_7_9dd44) -> id_line_6_7/1
  d_iq_line_9_4_block/1(Blockout_d_iq_line_9_4_61cd6) -> iq_line_9_4/1
  id_line_5_6/1 -> d_id_line_5_6_block/1(State_id_line_5_6_54864), d_iq_line_5_6_block/1(State_id_line_5_6_a16ef), id_bus_5_block/3(State_id_line_5_6_04a55), id_bus_6_block/2(State_id_line_5_6_c534c)
  id_bus_3_block/1(Blockout_id_bus_3_1118d) -> d_vd_bus_3_block/1(Alge_id_bus_3_78d4b)
  id_bus_8_block/1(Blockout_id_bus_8_d4ccc) -> d_vd_bus_8_block/1(Alge_id_bus_8_f6d08)
  iq_bus_7_block/1(Blockout_iq_bus_7_1b282) -> d_vq_bus_7_block/1(Alge_iq_bus_7_7a913)
  iq_bus_1_block/1(Blockout_iq_bus_1_79d62) -> d_vq_bus_1_block/1(Alge_iq_bus_1_2119b)
  id_bus_7_block/1(Blockout_id_bus_7_4fd6a) -> d_vd_bus_7_block/1(Alge_id_bus_7_e76ec)
  d_id_load_7_block/1(Blockout_d_id_load_7_5a75a) -> id_load_7/1
  iq_bus_6_block/1(Blockout_iq_bus_6_d8605) -> d_vq_bus_6_block/1(Alge_iq_bus_6_8b56a)
  id_line_4_5/1 -> id_bus_4_block/2(State_id_line_4_5_50091), d_iq_line_4_5_block/1(State_id_line_4_5_89819), d_id_line_4_5_block/1(State_id_line_4_5_63ee7), id_bus_5_block/2(State_id_line_4_5_6f8c4)
  id_bus_6_block/1(Blockout_id_bus_6_b1df2) -> d_vd_bus_6_block/1(Alge_id_bus_6_030aa)
  iq_bus_5_block/1(Blockout_iq_bus_5_9f39d) -> d_vq_bus_5_block/1(Alge_iq_bus_5_8f4e4)
  id_bus_5_block/1(Blockout_id_bus_5_7e5b8) -> d_vd_bus_5_block/1(Alge_id_bus_5_78beb)
  iq_bus_3_block/1(Blockout_iq_bus_3_7dfe9) -> d_vq_bus_3_block/1(Alge_iq_bus_3_59f2b)
  iq_line_9_4/1 -> d_id_line_9_4_block/2(State_iq_line_9_4_7582d), d_iq_line_9_4_block/2(State_iq_line_9_4_bf158), iq_bus_4_block/3(State_iq_line_9_4_15ad7), iq_bus_9_block/3(State_iq_line_9_4_aebff)
  d_iq_line_3_6_block/1(Blockout_d_iq_line_3_6_4acdf) -> iq_line_3_6/1
  vd_bus_4/1 -> d_id_line_1_4_block/3(State_vd_bus_4_b081e), d_id_line_4_5_block/3(State_vd_bus_4_38f30), d_id_line_9_4_block/3(State_vd_bus_4_3cbcb), d_vq_bus_4_block/2(State_vd_bus_4_2d95a)
  id_line_9_4/1 -> d_id_line_9_4_block/1(State_id_line_9_4_78432), d_iq_line_9_4_block/1(State_id_line_9_4_54433), id_bus_4_block/3(State_id_line_9_4_0046a), id_bus_9_block/3(State_id_line_9_4_b960f)
  vq_bus_8/1 -> d_iq_line_8_2_block/3(State_vq_bus_8_91184), d_iq_line_7_8_block/4(State_vq_bus_8_9183e), d_vd_bus_8_block/2(State_vq_bus_8_658d5), d_iq_line_8_9_block/3(State_vq_bus_8_a2731)
  d_vq_bus_8_block/1(Blockout_d_vq_bus_8_66a55) -> vq_bus_8/1
  id_load_7/1 -> id_bus_7_block/1(State_id_load_7_161b2), d_iq_load_7_block/1(State_id_load_7_916b5), d_id_load_7_block/1(State_id_load_7_50270)
  id_line_1_4/1 -> d_iq_line_1_4_block/1(State_id_line_1_4_24448), id_bus_4_block/1(State_id_line_1_4_2b5ff), id_bus_1_block/2(State_id_line_1_4_e0f83)
  id_bus_1_block/1(Blockout_id_bus_1_49cc3) -> d_vd_bus_1_block/1(Alge_id_bus_1_716c4)
  d_iq_line_6_7_block/1(Blockout_d_iq_line_6_7_4ed8f) -> iq_line_6_7/1
  d_vd_bus_7_block/1(Blockout_d_vd_bus_7_1b34a) -> vd_bus_7/1
  vd_bus_9/1 -> d_vq_bus_9_block/2(State_vd_bus_9_96e3e), d_id_load_9_block/3(State_vd_bus_9_f0529), d_id_line_8_9_block/4(State_vd_bus_9_a61c1), d_id_line_9_4_block/4(State_vd_bus_9_e3f3e)
  d_id_line_8_2_block/1(Blockout_d_id_line_8_2_9ff87) -> id_line_8_2/1
  d_vq_bus_9_block/1(Blockout_d_vq_bus_9_3fd84) -> vq_bus_9/1
  iq_load_9/1 -> d_id_load_9_block/2(State_iq_load_9_81910), d_iq_load_9_block/2(State_iq_load_9_12d39), iq_bus_9_block/1(State_iq_load_9_0a6dd)
  vd_bus_2/1 -> d_vq_bus_2_block/2(State_vd_bus_2_59719), vd_bus_2_out_block/1(State_vd_bus_2_38fae), d_id_line_8_2_block/2(State_vd_bus_2_94e9c)
  d_id_line_3_6_block/1(Blockout_d_id_line_3_6_a1287) -> id_line_3_6/1
  vd_bus_7/1 -> d_vq_bus_7_block/2(State_vd_bus_7_25da7), d_id_line_6_7_block/4(State_vd_bus_7_c0c3c), d_id_line_7_8_block/3(State_vd_bus_7_f48ac), d_id_load_7_block/3(State_vd_bus_7_8233e)
  iq_load_5/1 -> d_id_load_5_block/2(State_iq_load_5_85fa6), iq_bus_5_block/1(State_iq_load_5_a6c3f), d_iq_load_5_block/2(State_iq_load_5_1b5d6)
  id_line_8_9/1 -> id_bus_8_block/3(State_id_line_8_9_a20e3), d_id_line_8_9_block/1(State_id_line_8_9_36022), d_iq_line_8_9_block/1(State_id_line_8_9_f0140), id_bus_9_block/2(State_id_line_8_9_07115)
  vd_bus_3/1 -> d_vq_bus_3_block/2(State_vd_bus_3_a1107), d_id_line_3_6_block/2(State_vd_bus_3_54849), vd_bus_3_out_block/1(State_vd_bus_3_18f77)
  id_line_8_2/1 -> d_iq_line_8_2_block/1(State_id_line_8_2_ae494), id_bus_8_block/2(State_id_line_8_2_95418), id_bus_2_block/2(State_id_line_8_2_af6d6)
  iq_line_7_8/1 -> d_id_line_7_8_block/2(State_iq_line_7_8_44268), d_iq_line_7_8_block/2(State_iq_line_7_8_8dc14), iq_bus_7_block/3(State_iq_line_7_8_f10ed), iq_bus_8_block/1(State_iq_line_7_8_0fde7)
  iq_line_4_5/1 -> d_iq_line_4_5_block/2(State_iq_line_4_5_9f9c8), iq_bus_4_block/2(State_iq_line_4_5_efb88), iq_bus_5_block/2(State_iq_line_4_5_553d2), d_id_line_4_5_block/2(State_iq_line_4_5_db19e)
  iq_line_8_9/1 -> d_id_line_8_9_block/2(State_iq_line_8_9_f99c7), d_iq_line_8_9_block/2(State_iq_line_8_9_2d182), iq_bus_8_block/3(State_iq_line_8_9_635a9), iq_bus_9_block/2(State_iq_line_8_9_83b30)
  vd_bus_8/1 -> d_vq_bus_8_block/2(State_vd_bus_8_fb157), d_id_line_7_8_block/4(State_vd_bus_8_1c270), d_id_line_8_9_block/3(State_vd_bus_8_d11ac), d_id_line_8_2_block/3(State_vd_bus_8_dfb0e)
  iq_line_5_6/1 -> d_id_line_5_6_block/2(State_iq_line_5_6_98e26), iq_bus_5_block/3(State_iq_line_5_6_211b7), iq_bus_6_block/2(State_iq_line_5_6_6d34c), d_iq_line_5_6_block/2(State_iq_line_5_6_db011)
  iq_line_8_2/1 -> d_id_line_8_2_block/1(State_iq_line_8_2_cd298), iq_bus_2_block/2(State_iq_line_8_2_8ad2f), iq_bus_8_block/2(State_iq_line_8_2_e4d44)
  id_line_7_8/1 -> id_bus_8_block/1(State_id_line_7_8_11373), d_id_line_7_8_block/1(State_id_line_7_8_397f6), d_iq_line_7_8_block/1(State_id_line_7_8_f0710), id_bus_7_block/3(State_id_line_7_8_561bd)
  iq_line_6_7/1 -> d_id_line_6_7_block/2(State_iq_line_6_7_b228d), d_iq_line_6_7_block/2(State_iq_line_6_7_06b4f), iq_bus_6_block/3(State_iq_line_6_7_450ec), iq_bus_7_block/2(State_iq_line_6_7_cab3a)
  id_line_3_6/1 -> d_iq_line_3_6_block/1(State_id_line_3_6_9bf1f), id_bus_3_block/2(State_id_line_3_6_b321d), id_bus_6_block/1(State_id_line_3_6_3a667)
  iq_line_3_6/1 -> d_id_line_3_6_block/1(State_iq_line_3_6_4c99f), iq_bus_3_block/2(State_iq_line_3_6_4d41b), iq_bus_6_block/1(State_iq_line_3_6_ec9b9)
  vq_bus_9/1 -> d_vd_bus_9_block/2(State_vq_bus_9_34de9), d_iq_load_9_block/3(State_vq_bus_9_18995), d_iq_line_8_9_block/4(State_vq_bus_9_ce318), d_iq_line_9_4_block/4(State_vq_bus_9_c61bf)
  iq_line_1_4/1 -> d_id_line_1_4_block/1(State_iq_line_1_4_436b3), iq_bus_1_block/2(State_iq_line_1_4_7b28f), iq_bus_4_block/1(State_iq_line_1_4_47e2e)
  iq_load_7/1 -> d_id_load_7_block/2(State_iq_load_7_f0642), d_iq_load_7_block/2(State_iq_load_7_28c55), iq_bus_7_block/1(State_iq_load_7_d4d4f)
  vd_bus_5/1 -> d_vq_bus_5_block/2(State_vd_bus_5_3b4b0), d_id_line_4_5_block/4(State_vd_bus_5_ef8f6), d_id_line_5_6_block/3(State_vd_bus_5_724a2), d_id_load_5_block/3(State_vd_bus_5_7c4d9)
  id_load_5/1 -> d_id_load_5_block/1(State_id_load_5_57de7), d_iq_load_5_block/1(State_id_load_5_4850d), id_bus_5_block/1(State_id_load_5_a31e5)
  vq_bus_6/1 -> d_vd_bus_6_block/2(State_vq_bus_6_ee9a7), d_iq_line_3_6_block/3(State_vq_bus_6_81b3c), d_iq_line_5_6_block/4(State_vq_bus_6_0b890), d_iq_line_6_7_block/3(State_vq_bus_6_1b0a3)
  d_id_line_9_4_block/1(Blockout_d_id_line_9_4_e7536) -> id_line_9_4/1
  vq_bus_5/1 -> d_vd_bus_5_block/2(State_vq_bus_5_c24a2), d_iq_load_5_block/3(State_vq_bus_5_e375c), d_iq_line_4_5_block/4(State_vq_bus_5_9a267), d_iq_line_5_6_block/3(State_vq_bus_5_e8aa3)
  vq_bus_4/1 -> d_vd_bus_4_block/2(State_vq_bus_4_2d336), d_iq_line_1_4_block/3(State_vq_bus_4_1e5cd), d_iq_line_4_5_block/3(State_vq_bus_4_4222a), d_iq_line_9_4_block/3(State_vq_bus_4_44071)
  vd_bus_1/1 -> d_id_line_1_4_block/2(State_vd_bus_1_02b8d), vd_bus_1_out_block/1(State_vd_bus_1_5e32d), d_vq_bus_1_block/2(State_vd_bus_1_ddfcb)
  vq_bus_3/1 -> d_iq_line_3_6_block/2(State_vq_bus_3_40690), d_vd_bus_3_block/2(State_vq_bus_3_ecd7b), vq_bus_3_out_block/1(State_vq_bus_3_f0d02)
  d_vd_bus_3_block/1(Blockout_d_vd_bus_3_0aed6) -> vd_bus_3/1
  d_vq_bus_4_block/1(Blockout_d_vq_bus_4_587da) -> vq_bus_4/1
  d_vd_bus_9_block/1(Blockout_d_vd_bus_9_65c7e) -> vd_bus_9/1
  d_id_load_9_block/1(Blockout_d_id_load_9_4d2d3) -> id_load_9/1
  d_id_line_7_8_block/1(Blockout_d_id_line_7_8_bc37b) -> id_line_7_8/1
  d_iq_load_5_block/1(Blockout_d_iq_load_5_6b6fd) -> iq_load_5/1
  d_id_line_5_6_block/1(Blockout_d_id_line_5_6_f183f) -> id_line_5_6/1
  d_vq_bus_7_block/1(Blockout_d_vq_bus_7_d417b) -> vq_bus_7/1
  d_id_load_5_block/1(Blockout_d_id_load_5_8438f) -> id_load_5/1
  d_id_line_8_9_block/1(Blockout_d_id_line_8_9_70ad0) -> id_line_8_9/1
  d_vq_bus_2_block/1(Blockout_d_vq_bus_2_0966a) -> vq_bus_2/1
  d_vd_bus_1_block/1(Blockout_d_vd_bus_1_1c28f) -> vd_bus_1/1
  d_iq_line_1_4_block/1(Blockout_d_iq_line_1_4_76297) -> iq_line_1_4/1
  d_iq_line_4_5_block/1(Blockout_d_iq_line_4_5_94582) -> iq_line_4_5/1
  d_vd_bus_8_block/1(Blockout_d_vd_bus_8_439e3) -> vd_bus_8/1
  d_iq_line_5_6_block/1(Blockout_d_iq_line_5_6_4f412) -> iq_line_5_6/1
  d_vd_bus_6_block/1(Blockout_d_vd_bus_6_f68c6) -> vd_bus_6/1
  d_vd_bus_2_block/1(Blockout_d_vd_bus_2_5d58d) -> vd_bus_2/1
  d_iq_load_9_block/1(Blockout_d_iq_load_9_e3180) -> iq_load_9/1
  d_iq_line_7_8_block/1(Blockout_d_iq_line_7_8_9efcd) -> iq_line_7_8/1
  d_iq_line_8_9_block/1(Blockout_d_iq_line_8_9_92184) -> iq_line_8_9/1
  d_iq_load_7_block/1(Blockout_d_iq_load_7_45a74) -> iq_load_7/1
  d_vd_bus_5_block/1(Blockout_d_vd_bus_5_ea476) -> vd_bus_5/1
  d_vq_bus_1_block/1(Blockout_d_vq_bus_1_11663) -> vq_bus_1/1
  d_vq_bus_3_block/1(Blockout_d_vq_bus_3_e5e49) -> vq_bus_3/1
  d_vq_bus_5_block/1(Blockout_d_vq_bus_5_9db4d) -> vq_bus_5/1
  d_vq_bus_6_block/1(Blockout_d_vq_bus_6_8dd8e) -> vq_bus_6/1

== system case2/SG_D_1 ==
  v_d_SG_D_1 : Inport
  v_q_SG_D_1 : Inport  Port=2
  E_fd_SG_D_1 : Integrator  InitialCondition=2.102776684798402
  Px_1_SG_D_1 : Integrator  InitialCondition=0.0
  Px_2_SG_D_1 : Integrator  InitialCondition=0.0
  Px_3_SG_D_1 : Integrator  InitialCondition=7.15534538145087e-33
  R_f_SG_D_1 : Integrator  InitialCondition=14.196746589081783
  T_e_SG_D_1_block : Subsystem
  T_m_SG_D_1 : Integrator  InitialCondition=0.8089310711243431
  V_f_SG_D_1 : Integrator  InitialCondition=21.027766847984022
  d_E_fd_SG_D_1_block : Subsystem
  d_Px_1_SG_D_1_block : Subsystem
  d_Px_2_SG_D_1_block : Subsystem
  d_Px_3_SG_D_1_block : Subsystem
  d_R_f_SG_D_1_block : Subsystem
  d_T_m_SG_D_1_block : Subsystem
  d_V_f_SG_D_1_block : Subsystem
  d_psi_1d_SG_D_1_block : Subsystem
  d_psi_d_SG_D_1_block : Subsystem
  d_psi_fd_SG_D_1_block : Subsystem
  d_psi_gq_SG_D_1_block : Subsystem
  d_psi_kq_SG_D_1_block : Subsystem
  d_psi_q_SG_D_1_block : Subsystem
  d_theta_SG_D_1_block : Subsystem
  d_w_SG_D_1_block : Subsystem
  i_d_SG_D_1_block : Subsystem
  i_q_SG_D_1_block : Subsystem
  psi_1d_SG_D_1 : Integrator  InitialCondition=0.8174789299424732
  psi_d_SG_D_1 : Integrator  InitialCondition=0.7827411527842048
  psi_fd_SG_D_1 : Integrator  InitialCondition=0.9925573268201457
  psi_gq_SG_D_1 : Integrator  InitialCondition=0.3838518835887322
  psi_kq_SG_D_1 : Integrator  InitialCondition=-0.599768568107394
  psi_q_SG_D_1 : Integrator  InitialCondition=-0.6237593108316898
  theta_SG_D_1 : Integrator  InitialCondition=0.6725764701323949
  theta_SG_D_1_out_block : Subsystem
  w_SG_D_1 : Integrator  InitialCondition=376.99111843077515
  w_SG_D_1_out_block : Subsystem
  i_d_SG_D_1 : Outport
  i_q_SG_D_1 : Outport  Port=2
  T_e_SG_D_1 : Outport  Port=3
  w_SG_D_1_out : Outport  Port=4
  theta_SG_D_1_out : Outport  Port=5
  wires:
  d_Px_1_SG_D_1_block/1(Blockout_d_Px_1_SG_D_1_87980) -> Px_1_SG_D_1/1
  d_theta_SG_D_1_block/1(Blockout_d_theta_SG_D_1_14305) -> theta_SG_D_1/1
  V_f_SG_D_1/1 -> d_E_fd_SG_D_1_block/2(State_V_f_SG_D_1_bbd90), d_V_f_SG_D_1_block/14(State_V_f_SG_D_1_0d850)
  psi_kq_SG_D_1/1 -> d_psi_q_SG_D_1_block/2(State_psi_kq_SG_D_1_40857), d_psi_gq_SG_D_1_block/3(State_psi_kq_SG_D_1_4aba6), d_psi_gq_SG_D_1_block/5(State_psi_kq_SG_D_1_179c0), d_psi_kq_SG_D_1_block/2(State_psi_kq_SG_D_1_1e9b6), d_w_SG_D_1_block/5(State_psi_kq_SG_D_1_6b1f5), d_V_f_SG_D_1_block/10(State_psi_kq_SG_D_1_ede87), d_psi_kq_SG_D_1_block/4(State_psi_kq_SG_D_1_80b58), i_d_SG_D_1_block/2(State_psi_kq_SG_D_1_803a3), T_e_SG_D_1_block/3(State_psi_kq_SG_D_1_d34b9), d_psi_gq_SG_D_1_block/8(State_psi_kq_SG_D_1_a1242), i_q_SG_D_1_block/2(State_psi_kq_SG_D_1_9fa57)
  w_SG_D_1_out_block/1(Blockout_w_SG_D_1_out_1070a) -> w_SG_D_1_out/1
  w_SG_D_1/1 -> d_psi_q_SG_D_1_block/9(State_w_SG_D_1_591a9), d_psi_d_SG_D_1_block/9(State_w_SG_D_1_ca1da), d_V_f_SG_D_1_block/13(State_w_SG_D_1_6f530), d_w_SG_D_1_block/1(State_w_SG_D_1_09f18), d_theta_SG_D_1_block/1(State_w_SG_D_1_c2844), d_Px_2_SG_D_1_block/4(State_w_SG_D_1_63813), d_Px_1_SG_D_1_block/2(State_w_SG_D_1_30941), d_Px_3_SG_D_1_block/6(State_w_SG_D_1_cb78d), w_SG_D_1_out_block/1(State_w_SG_D_1_30d0f), d_V_f_SG_D_1_block/8(State_w_SG_D_1_ef9ca), d_T_m_SG_D_1_block/1(State_w_SG_D_1_af4aa)
  d_T_m_SG_D_1_block/1(Blockout_d_T_m_SG_D_1_1f476) -> T_m_SG_D_1/1
  d_Px_2_SG_D_1_block/1(Blockout_d_Px_2_SG_D_1_76795) -> Px_2_SG_D_1/1
  d_Px_3_SG_D_1_block/1(Blockout_d_Px_3_SG_D_1_a361e) -> Px_3_SG_D_1/1
  psi_gq_SG_D_1/1 -> d_psi_q_SG_D_1_block/1(State_psi_gq_SG_D_1_6c5f8), d_psi_gq_SG_D_1_block/1(State_psi_gq_SG_D_1_c4c61), d_psi_gq_SG_D_1_block/4(State_psi_gq_SG_D_1_a1618), d_psi_gq_SG_D_1_block/2(State_psi_gq_SG_D_1_a6c1d), d_psi_kq_SG_D_1_block/1(State_psi_gq_SG_D_1_c4f58), d_w_SG_D_1_block/4(State_psi_gq_SG_D_1_3c836), d_V_f_SG_D_1_block/9(State_psi_gq_SG_D_1_c85d3), i_d_SG_D_1_block/1(State_psi_gq_SG_D_1_57fbc), d_psi_gq_SG_D_1_block/7(State_psi_gq_SG_D_1_46c15), i_q_SG_D_1_block/1(State_psi_gq_SG_D_1_8309b), d_psi_kq_SG_D_1_block/3(State_psi_gq_SG_D_1_4c859), T_e_SG_D_1_block/2(State_psi_gq_SG_D_1_90d07)
  psi_fd_SG_D_1/1 -> d_psi_fd_SG_D_1_block/4(State_psi_fd_SG_D_1_817df), d_psi_fd_SG_D_1_block/2(State_psi_fd_SG_D_1_2c539), d_psi_fd_SG_D_1_block/7(State_psi_fd_SG_D_1_0d330), d_psi_fd_SG_D_1_block/10(State_psi_fd_SG_D_1_a3443), d_w_SG_D_1_block/10(State_psi_fd_SG_D_1_d4b67), d_V_f_SG_D_1_block/6(State_psi_fd_SG_D_1_5fa52), i_d_SG_D_1_block/7(State_psi_fd_SG_D_1_cd963), d_psi_1d_SG_D_1_block/5(State_psi_fd_SG_D_1_43baf), i_q_SG_D_1_block/7(State_psi_fd_SG_D_1_7071a), d_psi_1d_SG_D_1_block/2(State_psi_fd_SG_D_1_cc7fa), d_psi_d_SG_D_1_block/3(State_psi_fd_SG_D_1_71b08), T_e_SG_D_1_block/8(State_psi_fd_SG_D_1_72d5b)
  psi_d_SG_D_1/1 -> d_psi_fd_SG_D_1_block/6(State_psi_d_SG_D_1_5e4a1), d_psi_fd_SG_D_1_block/9(State_psi_d_SG_D_1_04628), d_psi_1d_SG_D_1_block/4(State_psi_d_SG_D_1_fa460), d_w_SG_D_1_block/3(State_psi_d_SG_D_1_d2513), d_V_f_SG_D_1_block/5(State_psi_d_SG_D_1_0f50c), d_V_f_SG_D_1_block/12(State_psi_d_SG_D_1_dda05), i_q_SG_D_1_block/6(State_psi_d_SG_D_1_d1dd7), d_psi_d_SG_D_1_block/2(State_psi_d_SG_D_1_7243c), d_w_SG_D_1_block/9(State_psi_d_SG_D_1_5c03b), T_e_SG_D_1_block/1(State_psi_d_SG_D_1_175f2), i_d_SG_D_1_block/6(State_psi_d_SG_D_1_bcca0), T_e_SG_D_1_block/7(State_psi_d_SG_D_1_deb78), d_psi_q_SG_D_1_block/8(State_psi_d_SG_D_1_19296)
  T_m_SG_D_1/1 -> d_T_m_SG_D_1_block/2(State_T_m_SG_D_1_b3cab), d_w_SG_D_1_block/2(State_T_m_SG_D_1_8218e)
  Px_1_SG_D_1/1 -> d_Px_3_SG_D_1_block/4(State_Px_1_SG_D_1_d5924), d_Px_2_SG_D_1_block/3(State_Px_1_SG_D_1_08e5e), d_Px_3_SG_D_1_block/5(State_Px_1_SG_D_1_8d63f), d_Px_2_SG_D_1_block/2(State_Px_1_SG_D_1_9c7e3), d_Px_1_SG_D_1_block/1(State_Px_1_SG_D_1_bfde0)
  v_d_SG_D_1/1 -> d_psi_q_SG_D_1_block/4(Input_v_d_SG_D_1_33d67), d_psi_d_SG_D_1_block/4(Input_v_d_SG_D_1_8f44e)
  v_q_SG_D_1/1 -> d_psi_d_SG_D_1_block/6(Input_v_q_SG_D_1_cfec8), d_psi_q_SG_D_1_block/6(Input_v_q_SG_D_1_717d9)
  psi_q_SG_D_1/1 -> d_psi_d_SG_D_1_block/8(State_psi_q_SG_D_1_21678), d_psi_q_SG_D_1_block/3(State_psi_q_SG_D_1_6bfdc), d_psi_gq_SG_D_1_block/6(State_psi_q_SG_D_1_4f03f), d_psi_gq_SG_D_1_block/9(State_psi_q_SG_D_1_9d78f), d_psi_kq_SG_D_1_block/5(State_psi_q_SG_D_1_7073d), d_V_f_SG_D_1_block/11(State_psi_q_SG_D_1_c5b3e), d_V_f_SG_D_1_block/7(State_psi_q_SG_D_1_18e5c), d_w_SG_D_1_block/7(State_psi_q_SG_D_1_8c671), i_d_SG_D_1_block/3(State_psi_q_SG_D_1_70a4f), T_e_SG_D_1_block/4(State_psi_q_SG_D_1_e9ca1), i_q_SG_D_1_block/3(State_psi_q_SG_D_1_72951), T_e_SG_D_1_block/5(State_psi_q_SG_D_1_1eaa9), d_w_SG_D_1_block/6(State_psi_q_SG_D_1_9a777)
  Px_2_SG_D_1/1 -> d_Px_3_SG_D_1_block/3(State_Px_2_SG_D_1_10f49), d_Px_2_SG_D_1_block/1(State_Px_2_SG_D_1_f9a06), d_Px_3_SG_D_1_block/2(State_Px_2_SG_D_1_26c88)
  theta_SG_D_1/1 -> d_psi_d_SG_D_1_block/5(State_theta_SG_D_1_4b996), d_psi_q_SG_D_1_block/5(State_theta_SG_D_1_0358b), d_psi_q_SG_D_1_block/7(State_theta_SG_D_1_cb754), i_d_SG_D_1_block/4(State_theta_SG_D_1_76dc5), i_d_SG_D_1_block/8(State_theta_SG_D_1_6bfd9), theta_SG_D_1_out_block/1(State_theta_SG_D_1_087cb), i_q_SG_D_1_block/8(State_theta_SG_D_1_754c0), i_q_SG_D_1_block/4(State_theta_SG_D_1_5ff93), d_psi_d_SG_D_1_block/7(State_theta_SG_D_1_e6cd3)
  d_E_fd_SG_D_1_block/1(Blockout_d_E_fd_SG_D_1_236a3) -> E_fd_SG_D_1/1
  psi_1d_SG_D_1/1 -> d_psi_fd_SG_D_1_block/5(State_psi_1d_SG_D_1_fa7db), d_psi_fd_SG_D_1_block/8(State_psi_1d_SG_D_1_ff3ca), d_psi_fd_SG_D_1_block/3(State_psi_1d_SG_D_1_28bae), d_psi_1d_SG_D_1_block/3(State_psi_1d_SG_D_1_c2340), d_w_SG_D_1_block/8(State_psi_1d_SG_D_1_38e11), d_V_f_SG_D_1_block/4(State_psi_1d_SG_D_1_653fa), i_d_SG_D_1_block/5(State_psi_1d_SG_D_1_4a4ce), d_psi_1d_SG_D_1_block/1(State_psi_1d_SG_D_1_9b7db), i_q_SG_D_1_block/5(State_psi_1d_SG_D_1_f4d32), T_e_SG_D_1_block/6(State_psi_1d_SG_D_1_6b7a6), d_psi_d_SG_D_1_block/1(State_psi_1d_SG_D_1_71504)
  d_R_f_SG_D_1_block/1(Blockout_d_R_f_SG_D_1_43b9e) -> R_f_SG_D_1/1
  d_V_f_SG_D_1_block/1(Blockout_d_V_f_SG_D_1_f2527) -> V_f_SG_D_1/1
  d_psi_d_SG_D_1_block/1(Blockout_d_psi_d_SG_D_1_ed5ed) -> psi_d_SG_D_1/1
  d_w_SG_D_1_block/1(Blockout_d_w_SG_D_1_3d550) -> w_SG_D_1/1
  T_e_SG_D_1_block/1(Blockout_T_e_SG_D_1_032d2) -> T_e_SG_D_1/1
  d_psi_1d_SG_D_1_block/1(Blockout_d_psi_1d_SG_D_1_2ff74) -> psi_1d_SG_D_1/1
  d_psi_q_SG_D_1_block/1(Blockout_d_psi_q_SG_D_1_0c4c1) -> psi_q_SG_D_1/1
  i_q_SG_D_1_block/1(Blockout_i_q_SG_D_1_07e0d) -> i_q_SG_D_1/1
  d_psi_kq_SG_D_1_block/1(Blockout_d_psi_kq_SG_D_1_aa20d) -> psi_kq_SG_D_1/1
  d_psi_gq_SG_D_1_block/1(Blockout_d_psi_gq_SG_D_1_ced27) -> psi_gq_SG_D_1/1
  i_d_SG_D_1_block/1(Blockout_i_d_SG_D_1_7a741) -> i_d_SG_D_1/1
  theta_SG_D_1_out_block/1(Blockout_theta_SG_D_1_out_5cdf6) -> theta_SG_D_1_out/1
  R_f_SG_D_1/1 -> d_R_f_SG_D_1_block/2(State_R_f_SG_D_1_c3db5), d_V_f_SG_D_1_block/2(State_R_f_SG_D_1_cec09)
  Px_3_SG_D_1/1 -> d_V_f_SG_D_1_block/3(State_Px_3_SG_D_1_d6039), d_Px_3_SG_D_1_block/1(State_Px_3_SG_D_1_70d34)
  E_fd_SG_D_1/1 -> d_E_fd_SG_D_1_block/1(State_E_fd_SG_D_1_3ff58), d_V_f_SG_D_1_block/1(State_E_fd_SG_D_1_db6b9), d_R_f_SG_D_1_block/1(State_E_fd_SG_D_1_fbe0c), d_psi_fd_SG_D_1_block/1(State_E_fd_SG_D_1_97de4)
  d_psi_fd_SG_D_1_block/1(Blockout_d_psi_fd_SG_D_1_670f9) -> psi_fd_SG_D_1/1
